simulink model "PhysicalLayerModel"  (R2013b)
settings: Solver=ode3  StartTime=0.0  StopTime=inf  RelTol=1e-3
model workspace (MAT data in the model file):
  CarrierFrequency = Simulink.Parameter
  CarrierFrequency.Value = 2600000
  CarrierFrequency.DataType = 'double'
  SampleTime = Simulink.Parameter
  SampleTime.Value = 1e-06
  SampleTime.DataType = 'double'
  SamplesPerFrame = Simulink.Parameter
  SamplesPerFrame.Value = 264
  SamplesPerFrame.DataType = 'double'
  M_ary = Simulink.Parameter
  M_ary.Value = 16
  M_ary.DataType = 'double'
  DelayParam = Simulink.Parameter
  DelayParam.Value = 2.66
  DelayParam.DataType = 'double'
  SNR = Simulink.Parameter
  SNR.Value = 30
  SNR.DataType = 'double'
  InputSignalPower = Simulink.Parameter
  InputSignalPower.Value = 1
  InputSignalPower.DataType = 'double'
  InterferanceFrequency = Simulink.Parameter
  InterferanceFrequency.Value = 0
  InterferanceFrequency.DataType = 'double'
  SymbolPhaseOffset = Simulink.Parameter
  SymbolPhaseOffset.Value = 0
  SymbolPhaseOffset.DataType = 'double'
  ModulationType = Simulink.Parameter
  ModulationType.Value = 0
  ModulationType.DataType = 'int8'
  SignalPower = Simulink.Parameter
  SignalPower.Value = 1
  SignalPower.DataType = 'double'
undefined symbols (not defined in the file): gcbh, rcfiltgaincompat
libraries: dspsrcs4 x8, simulink x8, commdigbbndpm3 x4, commfilt2 x4, commdigbbndam3 x4, commchan3 x2, commtimrec2 x2, dspsigops x2, commsink2 x2
settings Model: BufferReuse=off  Creator=The MathWorks Inc.  LastModifiedBy=Lucas
settings DataIOCC: SignalLoggingSaveFormat=ModelDataLogs  SaveOutput=off  SaveTime=off  SignalLoggingName=logsOut
settings OptimizationCC: OptimizeBlockIOStorage=off  BufferReuse=off  ExpressionFolding=off  ExpressionDepthLimit=2147483647  LocalBlockOutputs=off  InitFltsAndDblsToZero=on
settings DebuggingCC: SaveWithParameterizedLinksMsg=none  MergeDetectMultiDrivingBlocksExec=error  CheckExecutionContextPreStartOutputMsg=on  CheckExecutionContextRuntimeOutputMsg=on  SignalResolutionControl=TryResolveAllWithWarning  SolverPrmCheckMsg=none  InheritedTsInSrcMsg=none  MultiTaskDSMMsg=warning  MultiTaskCondExecSysMsg=none  StateNameClashWarn=warning
settings HardwareCC: ProdHWDeviceType=Specified  TargetLongLongMode=on  TargetIntDivRoundTo=Zero  TargetEndianess=LittleEndian  TargetHWDeviceType=MATLAB Host  ProdEqTarget=off
settings ModelReferenceCC: UpdateModelReferenceTargets=IfOutOfDate
settings RTWCC: GenCodeOnly=on  TemplateMakefile=RTW.MSVCBuild  Description=Create Visual C/C++ Solution File for Simulink Coder  ProcessScript=grt_make_rtw_hook  TargetLang=C++  IncludeERTFirstTime=on  CheckMdlBeforeBuild=Error
settings CodeAppCC: ForceParamTrailComments=on  MangleLength=5  MATLABSourceComments=on
settings GRTTargetCC: CodeReplacementLibrary=C89/C90 (ANSI)  MultiInstanceERTCode=on  GenerateAllocFcn=on  RTWCAPISignals=on  RTWCAPIParams=on

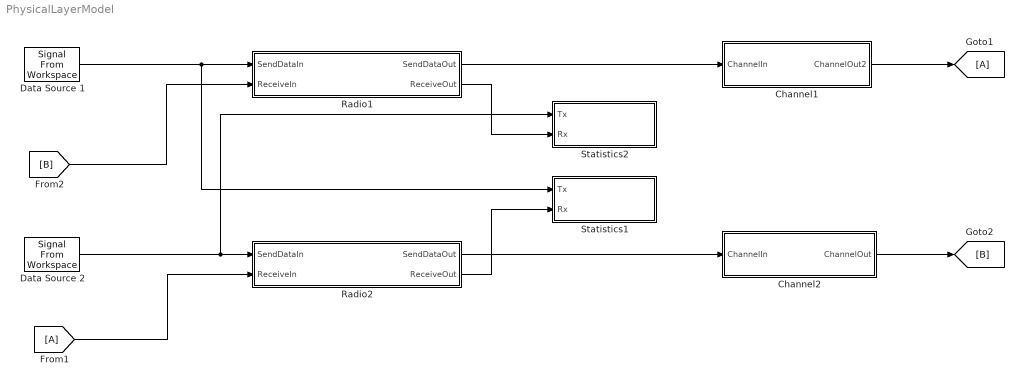
== system PhysicalLayerModel ==
  Channel1 : Subsystem  TreatAsAtomicUnit=on
      settings: RTWFcnNameOpts=Use subsystem name  RTWFileNameOpts=Use function name
  Channel2 : Subsystem  TreatAsAtomicUnit=on
      settings: RTWFcnNameOpts=Use subsystem name  RTWFileNameOpts=Use function name
  Data Source 1 : dspsrcs4/Signal From Workspace  X=data1  Ts=SampleTime  nsamps=SamplesPerFrame  OutputAfterFinalValue=Cyclic repetition  ignoreOrWarnInputAndFrameLengths=on
  Data Source 2 : dspsrcs4/Signal From Workspace  X=data2  Ts=SampleTime  nsamps=SamplesPerFrame  OutputAfterFinalValue=Cyclic repetition  ignoreOrWarnInputAndFrameLengths=on
  Radio1 : Subsystem
  Radio2 : Subsystem
  Statistics1 : Subsystem  TreatAsAtomicUnit=on
      settings: RTWFcnNameOpts=Use subsystem name  RTWFileNameOpts=Use function name
  Statistics2 : Subsystem  TreatAsAtomicUnit=on
      settings: RTWFcnNameOpts=Use subsystem name  RTWFileNameOpts=Use function name
  wires:
  Data Source 1/1 -> Statistics1/1(Tx), Radio1/1(SendDataIn)
  Channel1/1(ChannelOut2) -> [A]
  Radio1/1(SendDataOut) -> Channel1/1(ChannelIn)
  [B] -> Radio1/2(ReceiveIn)
  Radio2/1(SendDataOut) -> Channel2/1(ChannelIn)
  Data Source 2/1 -> Statistics2/1(Tx), Radio2/1(SendDataIn)
  Channel2/1(ChannelOut) -> [B]
  [A] -> Radio2/2(ReceiveIn)
  Radio2/2(ReceiveOut) -> Statistics1/2(Rx)
  Radio1/2(ReceiveOut) -> Statistics2/2(Rx)

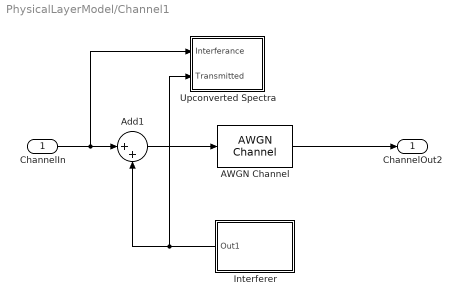
== system PhysicalLayerModel/Channel1 ==
  ChannelIn : Inport
  AWGN Channel : commchan3/AWGN Channel  InputProcessing=Columns as channels (frame based)  seed=67  noiseMode="Signal to noise ratio  (SNR)"  EbNodB=10  EsNodB=10  SNRdB=SNR  bitsPerSym=1  Ps=InputSignalPower  Tsym=1  variance=1
  Add1 : Sum  Inputs=|++
  Interferer : Subsystem  mask(Interference){nonlinOrder=3}
      mask prompts: nonlinOrder "Order of nonlinearity:"
      mask help: Generate out-of-band interference. Optionally process the interference with a third-order nonlinearity that creates an in-band harmonic.
      mask init:
      | if nonlinOrder == 1
      |     icontext = 'Interference\nwithout\nNonlinearity';
      | elseif nonlinOrder == 3
      |     icontext = 'Interference\nwith\nNonlinearity';
      | end
      mask Display: disp(icontext)
  Upconverted Spectra : Subsystem
      mask Display: disp('Upconverted\nSpectra')
  ChannelOut2 : Outport
  wires:
  Add1/1 -> AWGN Channel/1
  ChannelIn/1 -> Upconverted Spectra/1(Interferance), Add1/1
  AWGN Channel/1 -> ChannelOut2/1
  Interferer/1(Out1) -> Upconverted Spectra/2(Transmitted), Add1/2

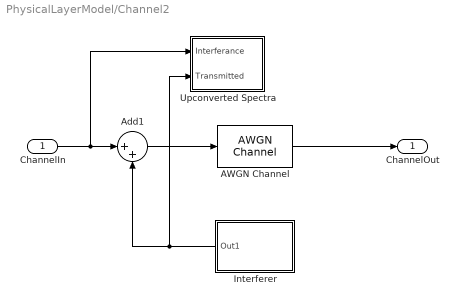
== system PhysicalLayerModel/Channel2 ==
  ChannelIn : Inport
  AWGN Channel : commchan3/AWGN Channel  InputProcessing=Columns as channels (frame based)  seed=67  noiseMode="Signal to noise ratio  (SNR)"  EbNodB=10  EsNodB=10  SNRdB=SNR  bitsPerSym=1  Ps=InputSignalPower  Tsym=1  variance=1
  Add1 : Sum  Inputs=|++
  Interferer : Subsystem  mask(Interference){nonlinOrder=3}
      mask prompts: nonlinOrder "Order of nonlinearity:"
      mask help: Generate out-of-band interference. Optionally process the interference with a third-order nonlinearity that creates an in-band harmonic.
      mask init:
      | if nonlinOrder == 1
      |     icontext = 'Interference\nwithout\nNonlinearity';
      | elseif nonlinOrder == 3
      |     icontext = 'Interference\nwith\nNonlinearity';
      | end
      mask Display: disp(icontext)
  Upconverted Spectra : Subsystem
      mask Display: disp('Upconverted\nSpectra')
  ChannelOut : Outport
  wires:
  Add1/1 -> AWGN Channel/1
  ChannelIn/1 -> Upconverted Spectra/1(Interferance), Add1/1
  AWGN Channel/1 -> ChannelOut/1
  Interferer/1(Out1) -> Upconverted Spectra/2(Transmitted), Add1/2

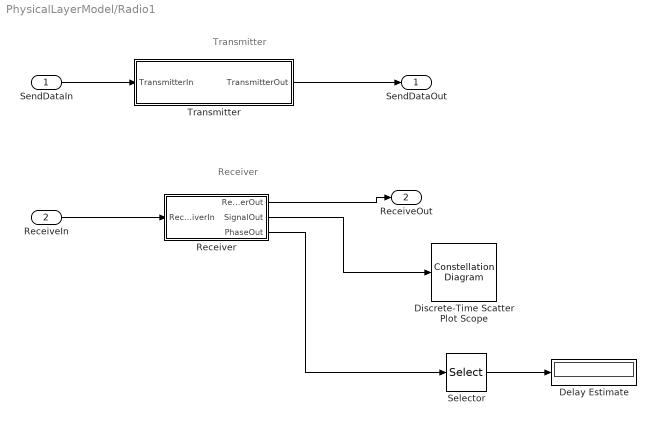
== system PhysicalLayerModel/Radio1 ==
  note: Transmitter
  note: Receiver
  SendDataIn : Inport
  ReceiveIn : Inport  Port=2
  Delay Estimate : Display
  Discrete-Time Scatter Plot Scope : ConstellationDiagram  Tag=ScatterPlot
      settings: CopyFcn=scopeextensions.ScopeBlock.onCoreBlockCopy(gcbh);  DeleteFcn=scopeextensions.ScopeBlock.callback(gcbh, 'onBlockDelete');  PreSaveFcn=scopeextensions.ScopeBlock.callback(gcbh, 'onModelSave');  NameChangeFcn=scopeextensions.ScopeBlock.callback(gcbh, 'onBlockRename');  DestroyFcn=scopeextensions.ScopeBlock.onBlockDestroy(gcbh)  CloseFcn=scopeextensions.ScopeBlock.callback(gcbh, 'onBlockClose');  PreDeleteFcn=scopeextensions.ScopeBlock.callback(gcbh, 'onBlockPreDelete');
  Receiver : Subsystem  TreatAsAtomicUnit=on
      settings: RTWFcnNameOpts=Use subsystem name  RTWFileNameOpts=Use function name
  Selector : Selector  InputPortWidth=SamplesPerFrame  IndexOptions=Index vector (dialog)  Indices=1  OutputSizes=1
  Transmitter : Subsystem  TreatAsAtomicUnit=on
      settings: RTWFcnNameOpts=Use subsystem name  RTWFileNameOpts=Use function name
  SendDataOut : Outport
  ReceiveOut : Outport  Port=2
  wires:
  SendDataIn/1 -> Transmitter/1(TransmitterIn)
  Transmitter/1(TransmitterOut) -> SendDataOut/1
  Receiver/1(ReceiverOut) -> ReceiveOut/1
  Selector/1 -> Delay Estimate/1
  Receiver/2(SignalOut) -> Discrete-Time Scatter Plot Scope/1
  Receiver/3(PhaseOut) -> Selector/1
  ReceiveIn/1 -> Receiver/1(ReceiverIn)

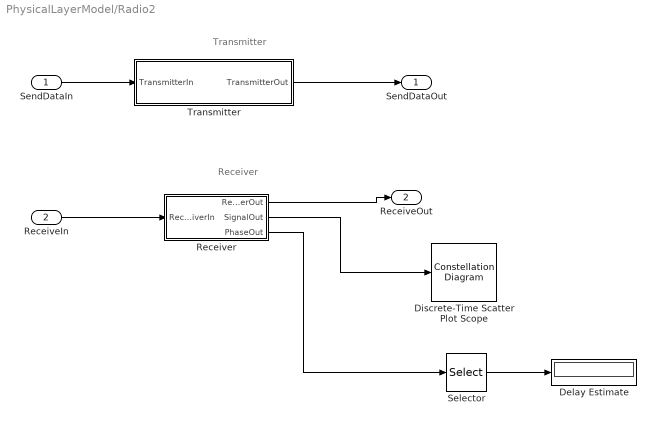
== system PhysicalLayerModel/Radio2 ==
  note: Transmitter
  note: Receiver
  SendDataIn : Inport
  ReceiveIn : Inport  Port=2
  Delay Estimate : Display
  Discrete-Time Scatter Plot Scope : ConstellationDiagram  Tag=ScatterPlot
      settings: CopyFcn=scopeextensions.ScopeBlock.onCoreBlockCopy(gcbh);  DeleteFcn=scopeextensions.ScopeBlock.callback(gcbh, 'onBlockDelete');  PreSaveFcn=scopeextensions.ScopeBlock.callback(gcbh, 'onModelSave');  NameChangeFcn=scopeextensions.ScopeBlock.callback(gcbh, 'onBlockRename');  DestroyFcn=scopeextensions.ScopeBlock.onBlockDestroy(gcbh)  CloseFcn=scopeextensions.ScopeBlock.callback(gcbh, 'onBlockClose');  PreDeleteFcn=scopeextensions.ScopeBlock.callback(gcbh, 'onBlockPreDelete');
  Receiver : Subsystem  TreatAsAtomicUnit=on
      settings: RTWFcnNameOpts=Use subsystem name  RTWFileNameOpts=Use function name
  Selector : Selector  InputPortWidth=SamplesPerFrame  IndexOptions=Index vector (dialog)  Indices=1  OutputSizes=1
  Transmitter : Subsystem  TreatAsAtomicUnit=on
      settings: RTWFcnNameOpts=Use subsystem name  RTWFileNameOpts=Use function name
  SendDataOut : Outport
  ReceiveOut : Outport  Port=2
  wires:
  SendDataIn/1 -> Transmitter/1(TransmitterIn)
  Transmitter/1(TransmitterOut) -> SendDataOut/1
  ReceiveIn/1 -> Receiver/1(ReceiverIn)
  Receiver/1(ReceiverOut) -> ReceiveOut/1
  Selector/1 -> Delay Estimate/1
  Receiver/2(SignalOut) -> Discrete-Time Scatter Plot Scope/1
  Receiver/3(PhaseOut) -> Selector/1

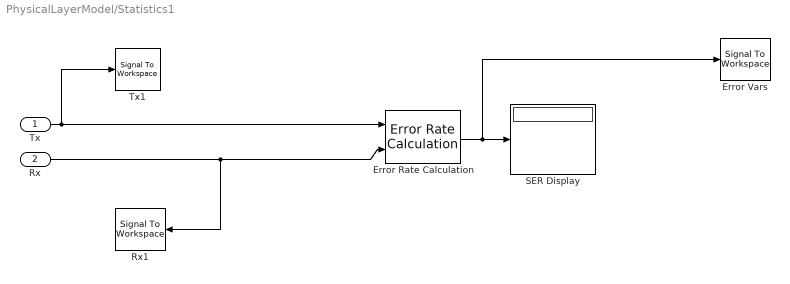
== system PhysicalLayerModel/Statistics1 ==
  Tx : Inport
  Rx : Inport  Port=2
  Error Rate Calculation : commsink2/Error Rate Calculation  N=8  st_delay=0  cp_mode=Entire frame  subframe=[]  PMode=Port  WsName=ErrorVec  RsMode2=off  stop=off  numErr=100  maxBits=1e6
  Error Vars : SignalToWorkspace  VariableName=ErrorVars1
      settings: CopyFcn=dspblkcopystw(gcbh);
  Rx1 : SignalToWorkspace  VariableName=Rx1
      settings: CopyFcn=dspblkcopystw(gcbh);
  SER Display : Display
  Tx1 : SignalToWorkspace  VariableName=Tx1
      settings: CopyFcn=dspblkcopystw(gcbh);
  wires:
  Error Rate Calculation/1 -> Error Vars/1, SER Display/1
  Tx/1 -> Tx1/1, Error Rate Calculation/1
  Rx/1 -> Rx1/1, Error Rate Calculation/2

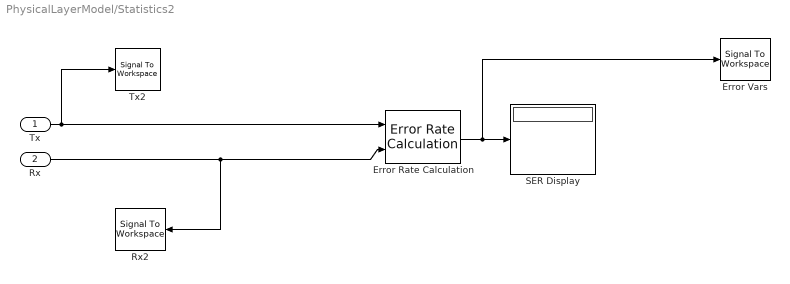
== system PhysicalLayerModel/Statistics2 ==
  Tx : Inport
  Rx : Inport  Port=2
  Error Rate Calculation : commsink2/Error Rate Calculation  N=8  st_delay=0  cp_mode=Entire frame  subframe=[]  PMode=Port  WsName=ErrorVec  RsMode2=off  stop=off  numErr=100  maxBits=1e6
  Error Vars : SignalToWorkspace  VariableName=ErrorVars2
      settings: CopyFcn=dspblkcopystw(gcbh);
  Rx2 : SignalToWorkspace  VariableName=Rx2
      settings: CopyFcn=dspblkcopystw(gcbh);
  SER Display : Display
  Tx2 : SignalToWorkspace  VariableName=Tx2
      settings: CopyFcn=dspblkcopystw(gcbh);
  wires:
  Error Rate Calculation/1 -> Error Vars/1, SER Display/1
  Tx/1 -> Tx2/1, Error Rate Calculation/1
  Rx/1 -> Rx2/1, Error Rate Calculation/2

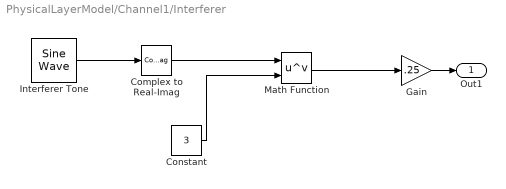
== system PhysicalLayerModel/Channel1/Interferer ==
  Complex to Real-Imag : ComplexToRealImag  Output=Real
  Constant : Constant  Value=3
  Gain : Gain  Gain=.25
  "Interferer Tone " : dspsrcs4/Sine Wave  Amplitude=1  Frequency=InterferanceFrequency  Phase=0  SampleMode=Discrete  OutComplex=Complex  CompMethod=Trigonometric fcn  TableSize=Speed  SampleTime=SampleTime/8  SamplesPerFrame=SamplesPerFrame * 8  ResetState=Restart at time zero  dataType=double  wordLen=16  udDataType=sfix(16)  fracBitsMode=Best precision  numFracBits=15  OutDataTypeStr=double  LastOutDataTypeStr=double
  Math Function : Math  Operator=pow  SaturateOnIntegerOverflow=on
  Out1 : Outport
  wires:
  Complex to Real-Imag/1 -> Math Function/1
  Constant/1 -> Math Function/2
  "Interferer Tone "/1 -> Complex to Real-Imag/1
  Math Function/1 -> Gain/1
  Gain/1 -> Out1/1

== system PhysicalLayerModel/Channel1/Upconverted Spectra ==
  Interferance : Inport
  Transmitted : Inport  Port=2
  Desired Signal and Interference : SpectrumAnalyzer
      settings: CopyFcn=scopeextensions.ScopeBlock.onCoreBlockCopy(gcbh);  DeleteFcn=scopeextensions.ScopeBlock.callback(gcbh, 'onBlockDelete');  PreSaveFcn=scopeextensions.ScopeBlock.callback(gcbh, 'onModelSave');  NameChangeFcn=scopeextensions.ScopeBlock.callback(gcbh, 'onBlockRename');  DestroyFcn=scopeextensions.ScopeBlock.onBlockDestroy(gcbh)  CloseFcn=scopeextensions.ScopeBlock.callback(gcbh, 'onBlockClose');  PreDeleteFcn=scopeextensions.ScopeBlock.callback(gcbh, 'onBlockPreDelete');
  Matrix Concatenation : Concatenate  Mode=Multidimensional array  ConcatenateDimension=2
  wires:
  Matrix Concatenation/1 -> Desired Signal and Interference/1
  Interferance/1 -> Matrix Concatenation/1
  Transmitted/1 -> Matrix Concatenation/2

== system PhysicalLayerModel/Channel2/Interferer ==
  Complex to Real-Imag : ComplexToRealImag  Output=Real
  Constant : Constant  Value=3
  Gain : Gain  Gain=.25
  "Interferer Tone " : dspsrcs4/Sine Wave  Amplitude=1  Frequency=InterferanceFrequency  Phase=0  SampleMode=Discrete  OutComplex=Complex  CompMethod=Trigonometric fcn  TableSize=Speed  SampleTime=SampleTime/8  SamplesPerFrame=SamplesPerFrame * 8  ResetState=Restart at time zero  dataType=double  wordLen=16  udDataType=sfix(16)  fracBitsMode=Best precision  numFracBits=15  OutDataTypeStr=double  LastOutDataTypeStr=double
  Math Function : Math  Operator=pow  SaturateOnIntegerOverflow=on
  Out1 : Outport
  wires:
  Complex to Real-Imag/1 -> Math Function/1
  Constant/1 -> Math Function/2
  "Interferer Tone "/1 -> Complex to Real-Imag/1
  Math Function/1 -> Gain/1
  Gain/1 -> Out1/1

== system PhysicalLayerModel/Channel2/Upconverted Spectra ==
  Interferance : Inport
  Transmitted : Inport  Port=2
  Desired Signal and Interference : SpectrumAnalyzer
      settings: CopyFcn=scopeextensions.ScopeBlock.onCoreBlockCopy(gcbh);  DeleteFcn=scopeextensions.ScopeBlock.callback(gcbh, 'onBlockDelete');  PreSaveFcn=scopeextensions.ScopeBlock.callback(gcbh, 'onModelSave');  NameChangeFcn=scopeextensions.ScopeBlock.callback(gcbh, 'onBlockRename');  DestroyFcn=scopeextensions.ScopeBlock.onBlockDestroy(gcbh)  CloseFcn=scopeextensions.ScopeBlock.callback(gcbh, 'onBlockClose');  PreDeleteFcn=scopeextensions.ScopeBlock.callback(gcbh, 'onBlockPreDelete');
  Matrix Concatenation : Concatenate  Mode=Multidimensional array  ConcatenateDimension=2
  wires:
  Matrix Concatenation/1 -> Desired Signal and Interference/1
  Interferance/1 -> Matrix Concatenation/1
  Transmitted/1 -> Matrix Concatenation/2

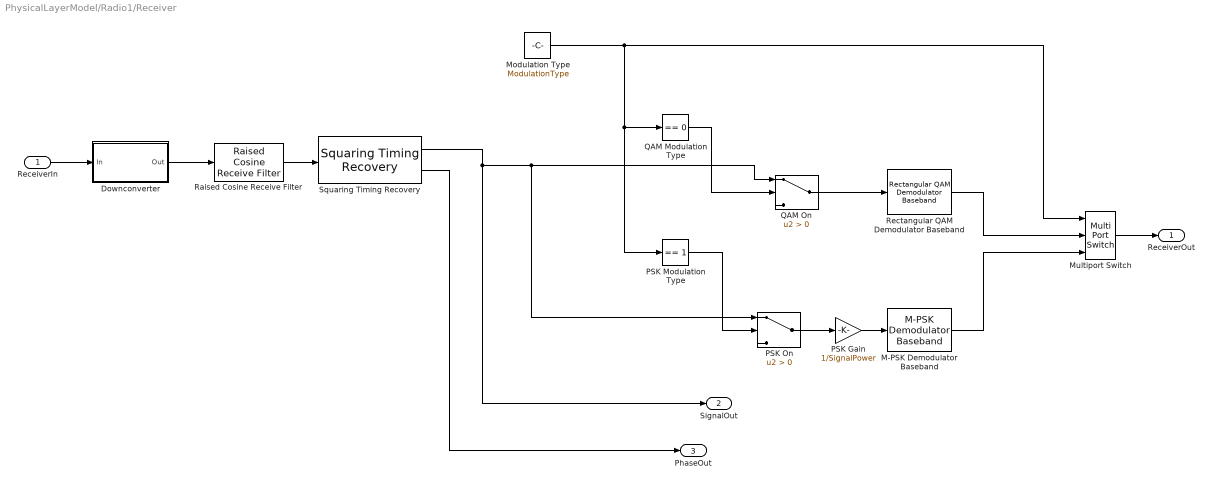
== system PhysicalLayerModel/Radio1/Receiver ==
  ReceiverIn : Inport
  Downconverter : Subsystem
      mask Display: disp('Downconverter')
  M-PSK Demodulator Baseband : commdigbbndpm3/M-PSK Demodulator Baseband  M=M_ary  Ph=pi/M_ary  Dec=Gray  Mapping=[0:7]  OutType=Integer  DecType=Hard decision  VarSource=Dialog  Variance=1  outDtype1=Inherit via internal rule  outDtype2=uint8  derotateFactorWordLen=16
  Modulation Type : Constant  Value=ModulationType
  Multiport Switch : MultiPortSwitch  DataPortOrder=Zero-based contiguous  Inputs=2
  PSK Gain : Gain  Gain=1/SignalPower
  PSK Modulation Type : simulink/Logic and Bit Operations/Compare To Constant  relop===  const=1  OutDataTypeStr=uint8
  PSK On : Switch  Criteria=u2 > Threshold
  QAM Modulation Type : simulink/Logic and Bit Operations/Compare To Constant  relop===  const=0  OutDataTypeStr=uint8
  QAM On : Switch  Criteria=u2 > Threshold
  Raised Cosine Receive Filter : commfilt2/Raised Cosine Receive Filter  filtType=Square root  N=8  filtSpan=2*(4)  currentFiltSpan=2*(4)  D=4  R=0.2  sampMode=Mute  saveAsFlag=0  rateMode=Downsampling  downFactor=1  downOffset=0  framing=Maintain input frame rate  InputProcessing=Columns as channels (frame based)  checkGain=Normalized  filterGain=rcfiltgaincompat(gcbh)  checkCoeff=off  variableName=rcRxFilt  launchFVT=off  roundingMode=Floor  overflowMode=off
  Rectangular QAM Demodulator Baseband : commdigbbndam3/Rectangular QAM Demodulator Baseband  M=M_ary  PowType=Min. distance between symbols  MinDist=SignalPower  AvgPow=1  PeakPow=1  Ph=SymbolPhaseOffset  Dec=Binary  Mapping=[0:15]  OutType=Integer  DecType=Hard decision  VarSource=Dialog  Variance=1  outDtype1=double  outDtype2=uint8  derotateFactorWordLen=16  denormFactorWordLen=16  prodOutWordLen=32  prodOutRoundingMode=Floor  prodOutOverflowMode=Wrap  sumWordLen=32
  Squaring Timing Recovery : commtimrec2/Squaring Timing Recovery  numSymb=SamplesPerFrame  sampPerSymb=8
  ReceiverOut : Outport
  SignalOut : Outport  Port=2
  PhaseOut : Outport  Port=3
  wires:
  Squaring Timing Recovery/2 -> PhaseOut/1
  Raised Cosine Receive Filter/1 -> Squaring Timing Recovery/1
  Downconverter/1(Out) -> Raised Cosine Receive Filter/1
  ReceiverIn/1 -> Downconverter/1(In)
  Rectangular QAM Demodulator Baseband/1 -> Multiport Switch/2
  M-PSK Demodulator Baseband/1 -> Multiport Switch/3
  Multiport Switch/1 -> ReceiverOut/1
  QAM On/1 -> Rectangular QAM Demodulator Baseband/1
  Squaring Timing Recovery/1 -> PSK On/1, QAM On/1, SignalOut/1
  Modulation Type/1 -> PSK Modulation Type/1, QAM Modulation Type/1, Multiport Switch/1
  QAM Modulation Type/1 -> QAM On/2
  PSK Modulation Type/1 -> PSK On/2
  PSK On/1 -> PSK Gain/1
  PSK Gain/1 -> M-PSK Demodulator Baseband/1

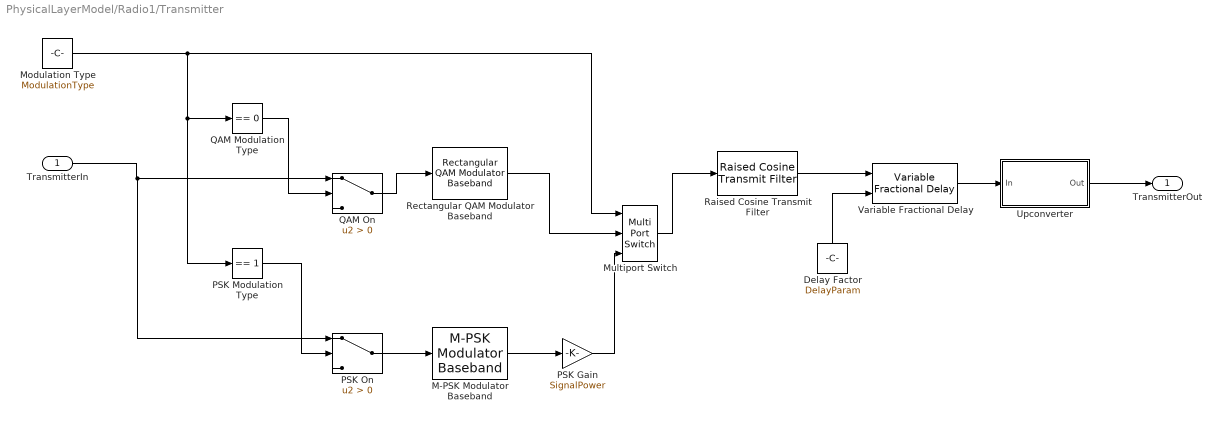
== system PhysicalLayerModel/Radio1/Transmitter ==
  TransmitterIn : Inport
  Delay Factor : Constant  Value=DelayParam
  M-PSK Modulator Baseband : commdigbbndpm3/M-PSK Modulator Baseband  M=M_ary  InType=Integer  Enc=Gray  Mapping=[0:7]  Ph=pi/M_ary  outDtype=double  outWordLen=16  outUDDataType=sfix(16)  outFracLenMode=Best precision  outFracLen=15
  Modulation Type : Constant  Value=ModulationType
  Multiport Switch : MultiPortSwitch  DataPortOrder=Zero-based contiguous  Inputs=2
  PSK Gain : Gain  Gain=SignalPower
  PSK Modulation Type : simulink/Logic and Bit Operations/Compare To Constant  relop===  const=1  OutDataTypeStr=uint8
  PSK On : Switch  Criteria=u2 > Threshold
  QAM Modulation Type : simulink/Logic and Bit Operations/Compare To Constant  relop===  const=0  OutDataTypeStr=uint8
  QAM On : Switch  Criteria=u2 > Threshold
  Raised Cosine Transmit Filter : commfilt2/Raised Cosine Transmit Filter  filtType=Square root  filtSpan=2*(4)  currentFiltSpan=2*(4)  D=(2*(4))/2  R=0.2  sampMode=Mute  saveAsFlag=0  N=8  framing=Enforce single-rate processing  InputProcessing=Columns as channels (frame based)  checkGain=Normalized  filterGain=rcfiltgaincompat(gcbh)  checkCoeff=off  variableName=rcTxFilt  launchFVT=off  roundingMode=Floor  overflowMode=off
  Rectangular QAM Modulator Baseband : commdigbbndam3/Rectangular QAM Modulator Baseband  M=M_ary  InType=Integer  Enc=Binary  Mapping=[0:15]  PowType=Min. distance between symbols  MinDist=SignalPower  AvgPow=1  PeakPow=1  Ph=SymbolPhaseOffset  outDtype=double  outWordLen=16  outUDDataType=sfix(16)  outFracLenMode=Best precision  outFracLen=15
  Upconverter : Subsystem
      mask Display: disp('Upconverter')
  Variable Fractional Delay : dspsigops/Variable Fractional Delay  mode=OBSOLETE  modeActive=Linear  dmax=4  InputProcessing=Columns as channels (frame based)  L=4  FarrowL=4  R=10  alpha=1  ic=0  fallbackFIR=Clip to the minimum value necessary for centered kernel  fallbackFarrow=Clip to the minimum value necessary for centered kernel  noDFT=off  roundingMode=Zero  overflowMode=off
  TransmitterOut : Outport
  wires:
  Delay Factor/1 -> Variable Fractional Delay/2
  Raised Cosine Transmit Filter/1 -> Variable Fractional Delay/1
  Variable Fractional Delay/1 -> Upconverter/1(In)
  Upconverter/1(Out) -> TransmitterOut/1
  Multiport Switch/1 -> Raised Cosine Transmit Filter/1
  Rectangular QAM Modulator Baseband/1 -> Multiport Switch/2
  Modulation Type/1 -> PSK Modulation Type/1, QAM Modulation Type/1, Multiport Switch/1
  TransmitterIn/1 -> PSK On/1, QAM On/1
  QAM On/1 -> Rectangular QAM Modulator Baseband/1
  PSK On/1 -> M-PSK Modulator Baseband/1
  QAM Modulation Type/1 -> QAM On/2
  PSK Modulation Type/1 -> PSK On/2
  M-PSK Modulator Baseband/1 -> PSK Gain/1
  PSK Gain/1 -> Multiport Switch/3

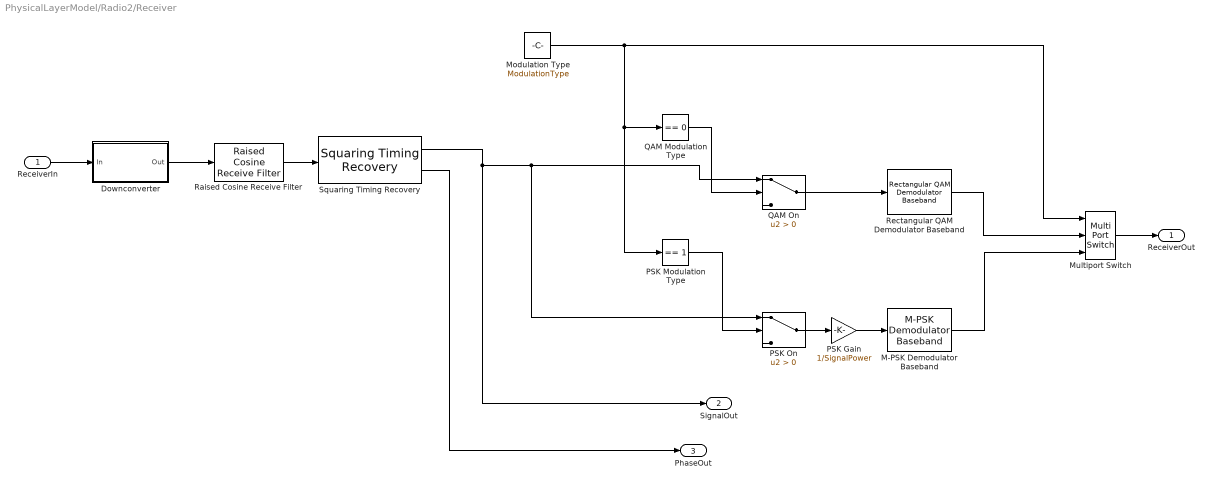
== system PhysicalLayerModel/Radio2/Receiver ==
  ReceiverIn : Inport
  Downconverter : Subsystem
      mask Display: disp('Downconverter')
  M-PSK Demodulator Baseband : commdigbbndpm3/M-PSK Demodulator Baseband  M=M_ary  Ph=pi/M_ary  Dec=Gray  Mapping=[0:7]  OutType=Integer  DecType=Hard decision  VarSource=Dialog  Variance=1  outDtype1=Inherit via internal rule  outDtype2=uint8  derotateFactorWordLen=16
  Modulation Type : Constant  Value=ModulationType
  Multiport Switch : MultiPortSwitch  DataPortOrder=Zero-based contiguous  Inputs=2
  PSK Gain : Gain  Gain=1/SignalPower
  PSK Modulation Type : simulink/Logic and Bit Operations/Compare To Constant  relop===  const=1  OutDataTypeStr=uint8
  PSK On : Switch  Criteria=u2 > Threshold
  QAM Modulation Type : simulink/Logic and Bit Operations/Compare To Constant  relop===  const=0  OutDataTypeStr=uint8
  QAM On : Switch  Criteria=u2 > Threshold
  Raised Cosine Receive Filter : commfilt2/Raised Cosine Receive Filter  filtType=Square root  N=8  filtSpan=2*(4)  currentFiltSpan=2*(4)  D=4  R=0.2  sampMode=Mute  saveAsFlag=0  rateMode=Downsampling  downFactor=1  downOffset=0  framing=Maintain input frame rate  InputProcessing=Columns as channels (frame based)  checkGain=Normalized  filterGain=rcfiltgaincompat(gcbh)  checkCoeff=off  variableName=rcRxFilt  launchFVT=off  roundingMode=Floor  overflowMode=off
  Rectangular QAM Demodulator Baseband : commdigbbndam3/Rectangular QAM Demodulator Baseband  M=M_ary  PowType=Min. distance between symbols  MinDist=SignalPower  AvgPow=1  PeakPow=1  Ph=SymbolPhaseOffset  Dec=Binary  Mapping=[0:15]  OutType=Integer  DecType=Hard decision  VarSource=Dialog  Variance=1  outDtype1=double  outDtype2=uint8  derotateFactorWordLen=16  denormFactorWordLen=16  prodOutWordLen=32  prodOutRoundingMode=Floor  prodOutOverflowMode=Wrap  sumWordLen=32
  Squaring Timing Recovery : commtimrec2/Squaring Timing Recovery  numSymb=SamplesPerFrame  sampPerSymb=8
  ReceiverOut : Outport
  SignalOut : Outport  Port=2
  PhaseOut : Outport  Port=3
  wires:
  Squaring Timing Recovery/2 -> PhaseOut/1
  Raised Cosine Receive Filter/1 -> Squaring Timing Recovery/1
  Downconverter/1(Out) -> Raised Cosine Receive Filter/1
  ReceiverIn/1 -> Downconverter/1(In)
  Rectangular QAM Demodulator Baseband/1 -> Multiport Switch/2
  Multiport Switch/1 -> ReceiverOut/1
  QAM On/1 -> Rectangular QAM Demodulator Baseband/1
  Squaring Timing Recovery/1 -> PSK On/1, QAM On/1, SignalOut/1
  Modulation Type/1 -> PSK Modulation Type/1, QAM Modulation Type/1, Multiport Switch/1
  QAM Modulation Type/1 -> QAM On/2
  PSK Modulation Type/1 -> PSK On/2
  M-PSK Demodulator Baseband/1 -> Multiport Switch/3
  PSK On/1 -> PSK Gain/1
  PSK Gain/1 -> M-PSK Demodulator Baseband/1

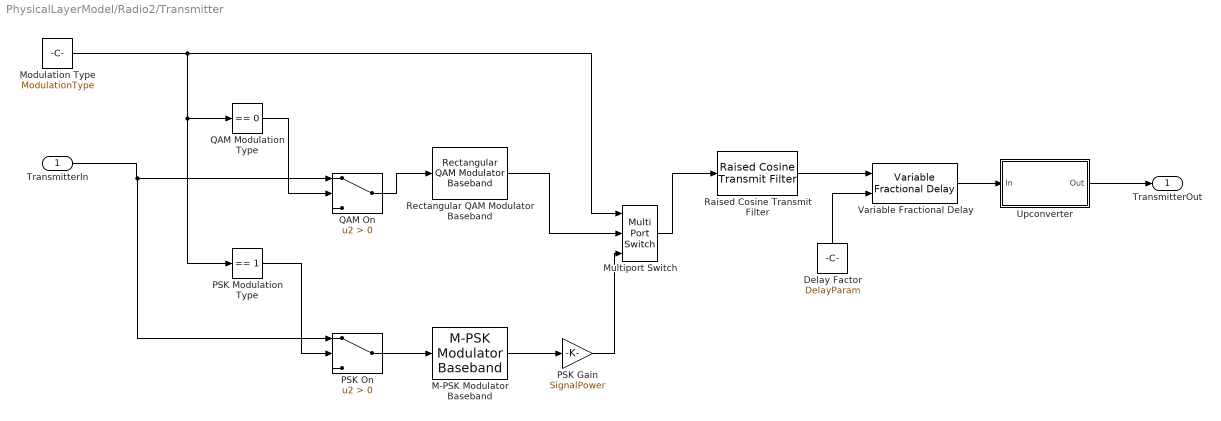
== system PhysicalLayerModel/Radio2/Transmitter ==
  TransmitterIn : Inport
  Delay Factor : Constant  Value=DelayParam
  M-PSK Modulator Baseband : commdigbbndpm3/M-PSK Modulator Baseband  M=M_ary  InType=Integer  Enc=Gray  Mapping=[0:7]  Ph=pi/M_ary  outDtype=double  outWordLen=16  outUDDataType=sfix(16)  outFracLenMode=Best precision  outFracLen=15
  Modulation Type : Constant  Value=ModulationType
  Multiport Switch : MultiPortSwitch  DataPortOrder=Zero-based contiguous  Inputs=2
  PSK Gain : Gain  Gain=SignalPower
  PSK Modulation Type : simulink/Logic and Bit Operations/Compare To Constant  relop===  const=1  OutDataTypeStr=uint8
  PSK On : Switch  Criteria=u2 > Threshold
  QAM Modulation Type : simulink/Logic and Bit Operations/Compare To Constant  relop===  const=0  OutDataTypeStr=uint8
  QAM On : Switch  Criteria=u2 > Threshold
  Raised Cosine Transmit Filter : commfilt2/Raised Cosine Transmit Filter  filtType=Square root  filtSpan=2*(4)  currentFiltSpan=2*(4)  D=4  R=0.2  sampMode=Mute  saveAsFlag=0  N=8  framing=Enforce single-rate processing  InputProcessing=Columns as channels (frame based)  checkGain=Normalized  filterGain=rcfiltgaincompat(gcbh)  checkCoeff=off  variableName=rcTxFilt  launchFVT=off  roundingMode=Floor  overflowMode=off
  Rectangular QAM Modulator Baseband : commdigbbndam3/Rectangular QAM Modulator Baseband  M=M_ary  InType=Integer  Enc=Binary  Mapping=[0:15]  PowType=Min. distance between symbols  MinDist=SignalPower  AvgPow=1  PeakPow=1  Ph=SymbolPhaseOffset  outDtype=double  outWordLen=16  outUDDataType=sfix(16)  outFracLenMode=Best precision  outFracLen=15
  Upconverter : Subsystem
      mask Display: disp('Upconverter')
  Variable Fractional Delay : dspsigops/Variable Fractional Delay  mode=OBSOLETE  modeActive=Linear  dmax=4  InputProcessing=Columns as channels (frame based)  L=4  FarrowL=4  R=10  alpha=1  ic=0  fallbackFIR=Clip to the minimum value necessary for centered kernel  fallbackFarrow=Clip to the minimum value necessary for centered kernel  noDFT=off  roundingMode=Zero  overflowMode=off
  TransmitterOut : Outport
  wires:
  Delay Factor/1 -> Variable Fractional Delay/2
  Raised Cosine Transmit Filter/1 -> Variable Fractional Delay/1
  Variable Fractional Delay/1 -> Upconverter/1(In)
  Upconverter/1(Out) -> TransmitterOut/1
  Multiport Switch/1 -> Raised Cosine Transmit Filter/1
  Rectangular QAM Modulator Baseband/1 -> Multiport Switch/2
  Modulation Type/1 -> PSK Modulation Type/1, QAM Modulation Type/1, Multiport Switch/1
  TransmitterIn/1 -> PSK On/1, QAM On/1
  QAM On/1 -> Rectangular QAM Modulator Baseband/1
  PSK On/1 -> M-PSK Modulator Baseband/1
  QAM Modulation Type/1 -> QAM On/2
  PSK Modulation Type/1 -> PSK On/2
  M-PSK Modulator Baseband/1 -> PSK Gain/1
  PSK Gain/1 -> Multiport Switch/3

== system PhysicalLayerModel/Radio1/Receiver/Downconverter ==
  In : Inport
  Conjugate : Math  Operator=conj  SaturateOnIntegerOverflow=on
  Downfrequency Oscillator : dspsrcs4/Sine Wave  Amplitude=1  Frequency=CarrierFrequency  Phase=0  SampleMode=Discrete  OutComplex=Complex  CompMethod=Trigonometric fcn  TableSize=Speed  SampleTime=SampleTime/8  SamplesPerFrame=SamplesPerFrame * 8  ResetState=Restart at time zero  dataType=double  wordLen=16  udDataType=sfix(16)  fracBitsMode=Best precision  numFracBits=15  OutDataTypeStr=double  LastOutDataTypeStr=double
  Product1 : Product  RndMeth=Zero
  Out : Outport
  wires:
  Conjugate/1 -> Product1/1
  Product1/1 -> Out/1
  In/1 -> Product1/2
  Downfrequency Oscillator/1 -> Conjugate/1

== system PhysicalLayerModel/Radio1/Transmitter/Upconverter ==
  In : Inport
  Complex to Real-Imag : ComplexToRealImag  Output=Real
  Product : Product  RndMeth=Zero
  Upfrequency Oscillator : dspsrcs4/Sine Wave  Amplitude=2  Frequency=CarrierFrequency  Phase=0  SampleMode=Discrete  OutComplex=Complex  CompMethod=Trigonometric fcn  TableSize=Speed  SampleTime=SampleTime/8  SamplesPerFrame=SamplesPerFrame * 8  ResetState=Restart at time zero  dataType=double  wordLen=16  udDataType=sfix(16)  fracBitsMode=Best precision  numFracBits=15  OutDataTypeStr=double  LastOutDataTypeStr=double
  Out : Outport
  wires:
  Complex to Real-Imag/1 -> Out/1
  Product/1 -> Complex to Real-Imag/1
  Upfrequency Oscillator/1 -> Product/2
  In/1 -> Product/1

== system PhysicalLayerModel/Radio2/Receiver/Downconverter ==
  In : Inport
  Conjugate : Math  Operator=conj  SaturateOnIntegerOverflow=on
  Downfrequency Oscillator : dspsrcs4/Sine Wave  Amplitude=1  Frequency=CarrierFrequency  Phase=0  SampleMode=Discrete  OutComplex=Complex  CompMethod=Trigonometric fcn  TableSize=Speed  SampleTime=SampleTime/8  SamplesPerFrame=SamplesPerFrame * 8  ResetState=Restart at time zero  dataType=double  wordLen=16  udDataType=sfix(16)  fracBitsMode=Best precision  numFracBits=15  OutDataTypeStr=double  LastOutDataTypeStr=double
  Product1 : Product  RndMeth=Zero
  Out : Outport
  wires:
  Conjugate/1 -> Product1/1
  Product1/1 -> Out/1
  In/1 -> Product1/2
  Downfrequency Oscillator/1 -> Conjugate/1

== system PhysicalLayerModel/Radio2/Transmitter/Upconverter ==
  In : Inport
  Complex to Real-Imag : ComplexToRealImag  Output=Real
  Product : Product  RndMeth=Zero
  Upfrequency Oscillator : dspsrcs4/Sine Wave  Amplitude=2  Frequency=CarrierFrequency  Phase=0  SampleMode=Discrete  OutComplex=Complex  CompMethod=Trigonometric fcn  TableSize=Speed  SampleTime=SampleTime/8  SamplesPerFrame=SamplesPerFrame * 8  ResetState=Restart at time zero  dataType=double  wordLen=16  udDataType=sfix(16)  fracBitsMode=Best precision  numFracBits=15  OutDataTypeStr=double  LastOutDataTypeStr=double
  Out : Outport
  wires:
  Complex to Real-Imag/1 -> Out/1
  Product/1 -> Complex to Real-Imag/1
  Upfrequency Oscillator/1 -> Product/2
  In/1 -> Product/1
